simulink subsystem "nonlinear_model"  (R2026a)
settings: Solver=VariableStepAuto
values from neighbouring files (symbols this model uses):
  b = P.b    [init_workspace.m]
  d = P.d    [init_workspace.m]
  g = P.g    [init_workspace.m]
  m = P.m    [init_workspace.m]
undefined symbols (not defined in the file or in its folder): P
settings Model: Creator=Kiril  LastModifiedBy=Kiril

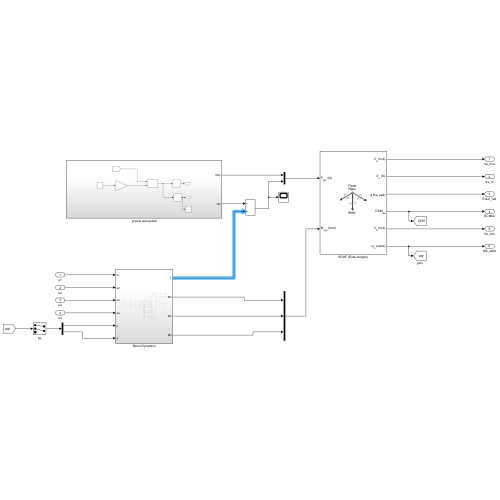
[thumbnail: Simulink's stored preview of the top-level diagram]
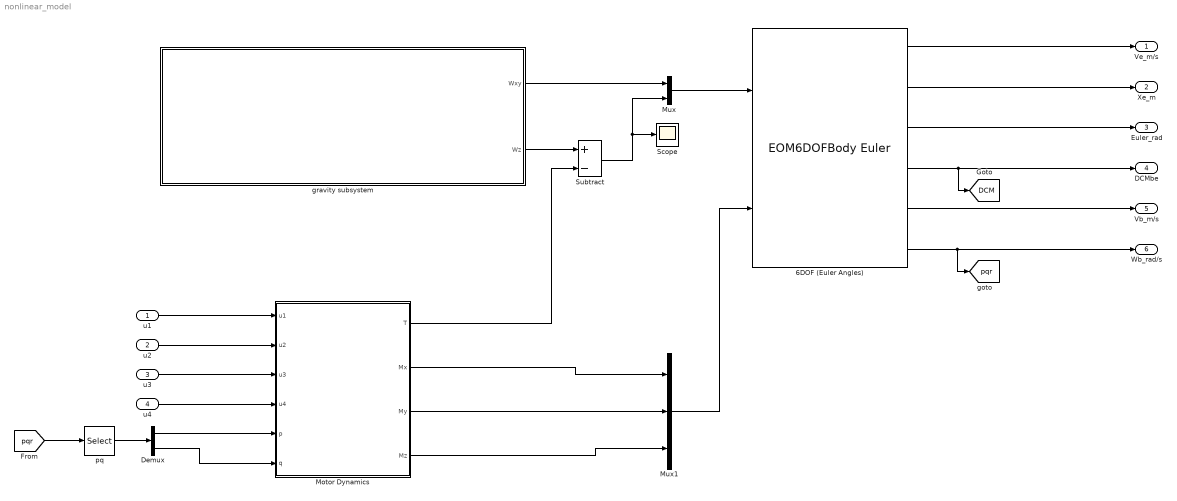
== system nonlinear_model ==
  u1 : Inport
  u2 : Inport  Port=2
  u3 : Inport  Port=3
  u4 : Inport  Port=4
  " gravity subsystem" : Subsystem
  6DOF (Euler Angles) : EOM6DOFBodyEuler  xme_0=Sim.Initial_Position  Vm_0=Sim.Initial_Velocity_Body  eul_0=Sim.Initial_Euler_Angles_Rad  pm_0=Sim.Initial_Body_Angular_Rates_Rads  mass_0=m  inertia=P.I
  Demux : Demux  Outputs=2
  Motor Dynamics : Subsystem
  Mux : Mux  Inputs=2
  Mux1 : Mux  Inputs=3
  Scope : Scope
      settings: ActiveDisplayYMinimum=-2.4563987435086156  ActiveDisplayYMaximum=16.534238683325494  DataLoggingVariableName=ScopeData9
  Subtract : Sum  Inputs=+-
  pq : Selector  InputPortWidth=3  IndexOptions=Index vector (dialog)  Indices=[1 2]  OutputSizes=1
  Ve_m/s : Outport
  Xe_m : Outport  Port=2
  Euler_rad : Outport  Port=3
  DCMbe : Outport  Port=4
  Vb_m/s : Outport  Port=5
  Wb_rad/s : Outport  Port=6
  tag scope: DCM=global, pqr=global
  wires:
  u1/1 -> Motor Dynamics/1(u1)
  u2/1 -> Motor Dynamics/2(u2)
  u3/1 -> Motor Dynamics/3(u3)
  u4/1 -> Motor Dynamics/4(u4)
  [pqr] -> pq/1
  pq/1 -> Demux/1
  Demux/1 -> Motor Dynamics/5(p)
  Demux/2 -> Motor Dynamics/6(q)
  6DOF (Euler Angles)/4 -> DCMbe/1, [DCM]
  " gravity subsystem"/2(Wz) -> Subtract/1
  Motor Dynamics/1(T) -> Subtract/2
  Mux/1 -> 6DOF (Euler Angles)/1
  " gravity subsystem"/1(Wxy) -> Mux/1
  Subtract/1 -> Mux/2, Scope/1
  Motor Dynamics/2(Mx) -> Mux1/1
  Motor Dynamics/3(My) -> Mux1/2
  Motor Dynamics/4(Mz) -> Mux1/3
  Mux1/1 -> 6DOF (Euler Angles)/2
  6DOF (Euler Angles)/1 -> Ve_m/s/1
  6DOF (Euler Angles)/2 -> Xe_m/1
  6DOF (Euler Angles)/3 -> Euler_rad/1
  6DOF (Euler Angles)/5 -> Vb_m/s/1
  6DOF (Euler Angles)/6 -> Wb_rad/s/1, [pqr]

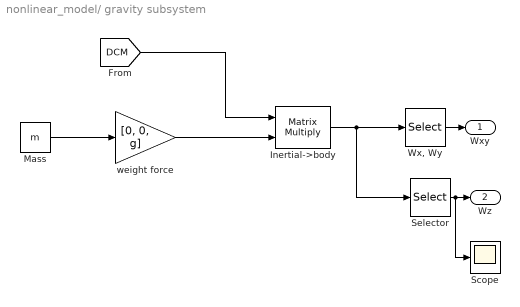
== system nonlinear_model/ gravity subsystem ==
  Inertial->body : Product  Multiplication=Matrix(*)
  Mass : Constant  Value=m
  Scope : Scope
      settings: ActiveDisplayYMinimum=4.3832987568990287  ActiveDisplayYMaximum=18.155212738596219  DataLoggingVariableName=ScopeData10
  Selector : Selector  InputPortWidth=3  IndexOptions=Index vector (dialog)  Indices=3  OutputSizes=1
  "Wx, Wy" : Selector  InputPortWidth=3  IndexOptions=Index vector (dialog)  Indices=[1 2]  OutputSizes=1
  weight force : Gain  Gain=[0, 0, g]
  Wxy : Outport
  Wz : Outport  Port=2
  wires:
  Inertial->body/1 -> Selector/1, "Wx, Wy"/1
  Mass/1 -> weight force/1
  [DCM] -> Inertial->body/1
  Selector/1 -> Wz/1, Scope/1
  weight force/1 -> Inertial->body/2
  "Wx, Wy"/1 -> Wxy/1

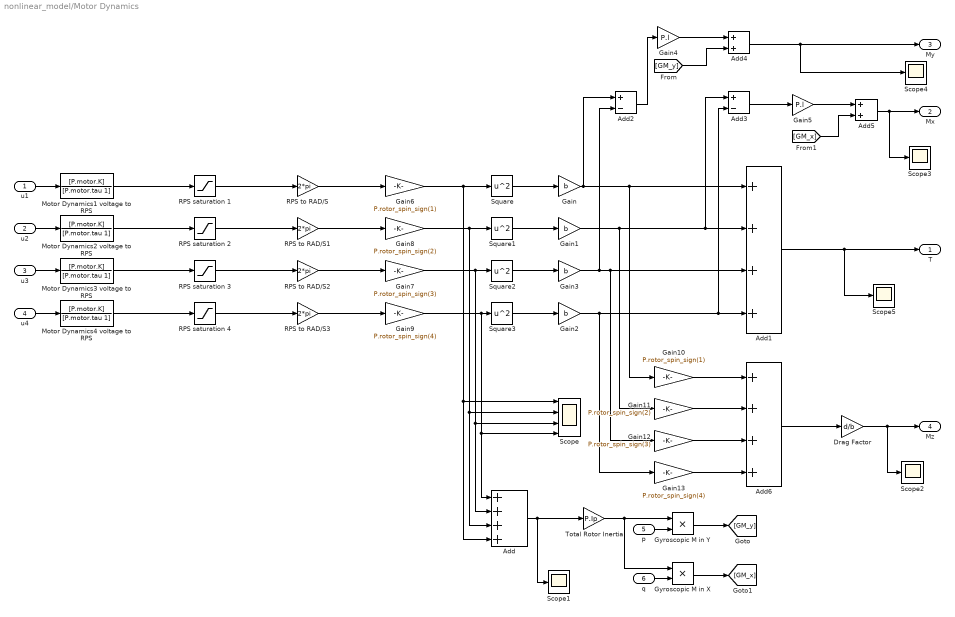
== system nonlinear_model/Motor Dynamics ==
  u1 : Inport
  u2 : Inport  Port=2
  u3 : Inport  Port=3
  u4 : Inport  Port=4
  p : Inport  Port=5
  q : Inport  Port=6
  Add : Sum  Inputs=++++
  Add1 : Sum  Inputs=++++
  Add2 : Sum  Inputs=+-
  Add3 : Sum  Inputs=+-
  Add4 : Sum
  Add5 : Sum
  Add6 : Sum  Inputs=++++
  Drag Factor : Gain  Gain=d/b
  Gain{,1..3} (4 alike) : Gain  Gain=b
  Gain10 : Gain  Gain=P.rotor_spin_sign(1)
  Gain11 : Gain  Gain=P.rotor_spin_sign(2)
  Gain12 : Gain  Gain=P.rotor_spin_sign(3)
  Gain13 : Gain  Gain=P.rotor_spin_sign(4)
  Gain4 : Gain  Gain=P.l
  Gain5 : Gain  Gain=P.l
  Gain6 : Gain  Gain=P.rotor_spin_sign(1)
  Gain7 : Gain  Gain=P.rotor_spin_sign(3)
  Gain8 : Gain  Gain=P.rotor_spin_sign(2)
  Gain9 : Gain  Gain=P.rotor_spin_sign(4)
  Gyroscopic M in X : Product
  Gyroscopic M in Y : Product
  Motor Dynamics1 voltage to RPS : TransferFcn  Numerator=[P.motor.K]  Denominator=[P.motor.tau 1]
  Motor Dynamics2 voltage to RPS : TransferFcn  Numerator=[P.motor.K]  Denominator=[P.motor.tau 1]
  Motor Dynamics3 voltage to RPS : TransferFcn  Numerator=[P.motor.K]  Denominator=[P.motor.tau 1]
  Motor Dynamics4 voltage to RPS : TransferFcn  Numerator=[P.motor.K]  Denominator=[P.motor.tau 1]
  RPS saturation {1..4} (4 alike) : Saturate  UpperLimit=P.motor.rps_max  LowerLimit=P.motor.rps_min
  RPS to RAD/S{,1..3} (4 alike) : Gain  Gain=2*pi
  Scope : Scope  NumInputPorts=4
      settings: ActiveDisplayYMinimum=368.29331773736612  ActiveDisplayYMaximum=598.48419665267454  DataLoggingVariableName=ScopeData3
  Scope{1..5} (5 alike) : Scope
      Scope1 settings: ActiveDisplayYMinimum=-1  ActiveDisplayYMaximum=1  DataLoggingVariableName=ScopeData5
      Scope2 settings: ActiveDisplayYMinimum=-1  ActiveDisplayYMaximum=1  DataLoggingVariableName=ScopeData4
      Scope3 settings: ActiveDisplayYMinimum=-1  ActiveDisplayYMaximum=1  DataLoggingVariableName=ScopeData6
      Scope4 settings: ActiveDisplayYMinimum=-1  ActiveDisplayYMaximum=1  DataLoggingVariableName=ScopeData7
      Scope5 settings: ActiveDisplayYMinimum=12.35857291589145  ActiveDisplayYMaximum=13.944979636858571  DataLoggingVariableName=ScopeData8
  Square{,1..3} (4 alike) : Math  Operator=square
  Total Rotor Inertia : Gain  Gain=P.Ip
  T : Outport
  Mx : Outport  Port=2
  My : Outport  Port=3
  Mz : Outport  Port=4
  wires:
  u1/1 -> Motor Dynamics1 voltage to RPS/1
  u2/1 -> Motor Dynamics2 voltage to RPS/1
  u3/1 -> Motor Dynamics3 voltage to RPS/1
  u4/1 -> Motor Dynamics4 voltage to RPS/1
  Add/1 -> Total Rotor Inertia/1, Scope1/1
  p/1 -> Gyroscopic M in Y/2
  Total Rotor Inertia/1 -> Gyroscopic M in X/1, Gyroscopic M in Y/1
  q/1 -> Gyroscopic M in X/2
  Gyroscopic M in Y/1 -> [GM_y]
  Gyroscopic M in X/1 -> [GM_x]
  Square/1 -> Gain/1
  Square1/1 -> Gain1/1
  Square2/1 -> Gain3/1
  Square3/1 -> Gain2/1
  Add1/1 -> T/1, Scope5/1
  Add2/1 -> Gain4/1
  Gain4/1 -> Add4/1
  [GM_y] -> Add4/2
  Add3/1 -> Gain5/1
  Gain5/1 -> Add5/1
  [GM_x] -> Add5/2
  Add6/1 -> Drag Factor/1
  Add5/1 -> Mx/1, Scope3/1
  Add4/1 -> My/1, Scope4/1
  Drag Factor/1 -> Mz/1, Scope2/1
  Gain6/1 -> Add/4, Scope/1, Square/1
  Gain7/1 -> Square2/1, Add/2, Scope/3
  Gain8/1 -> Add/3, Scope/2, Square1/1
  Gain9/1 -> Add/1, Scope/4, Square3/1
  Gain/1 -> Add2/1, Gain10/1, Add1/1
  Gain1/1 -> Gain11/1, Add3/1, Add1/2
  Gain3/1 -> Add2/2, Gain12/1, Add1/3
  Gain2/1 -> Gain13/1, Add3/2, Add1/4
  Gain10/1 -> Add6/1
  Gain11/1 -> Add6/2
  Gain12/1 -> Add6/3
  Gain13/1 -> Add6/4
  RPS to RAD/S/1 -> Gain6/1
  RPS to RAD/S1/1 -> Gain8/1
  RPS to RAD/S2/1 -> Gain7/1
  RPS to RAD/S3/1 -> Gain9/1
  RPS saturation 4/1 -> RPS to RAD/S3/1
  Motor Dynamics4 voltage to RPS/1 -> RPS saturation 4/1
  RPS saturation 3/1 -> RPS to RAD/S2/1
  Motor Dynamics3 voltage to RPS/1 -> RPS saturation 3/1
  RPS saturation 2/1 -> RPS to RAD/S1/1
  Motor Dynamics2 voltage to RPS/1 -> RPS saturation 2/1
  RPS saturation 1/1 -> RPS to RAD/S/1
  Motor Dynamics1 voltage to RPS/1 -> RPS saturation 1/1
